simulink model "practia1"  (R2024b)
settings: Solver=VariableStepAuto  StartTime=0.0  StopTime=20  MaxStep=0.01  RelTol=1e-3
InitFcn:
  | ip = 0.0079;
  | Mc = 0.7031;
  | Lp = 0.3302;
  | Mp = 0.23;
  | Fc = 0;
  | Beq = 4.3;
  | g = 9.81;
  | Bp = 0.0024;
settings Model: LastModifiedBy=52332

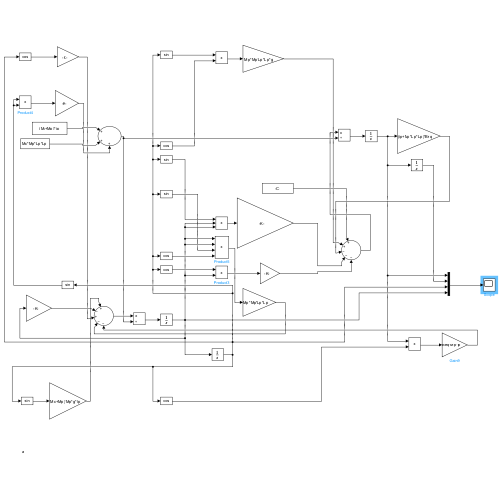
[thumbnail: Simulink's stored preview of the top-level diagram]
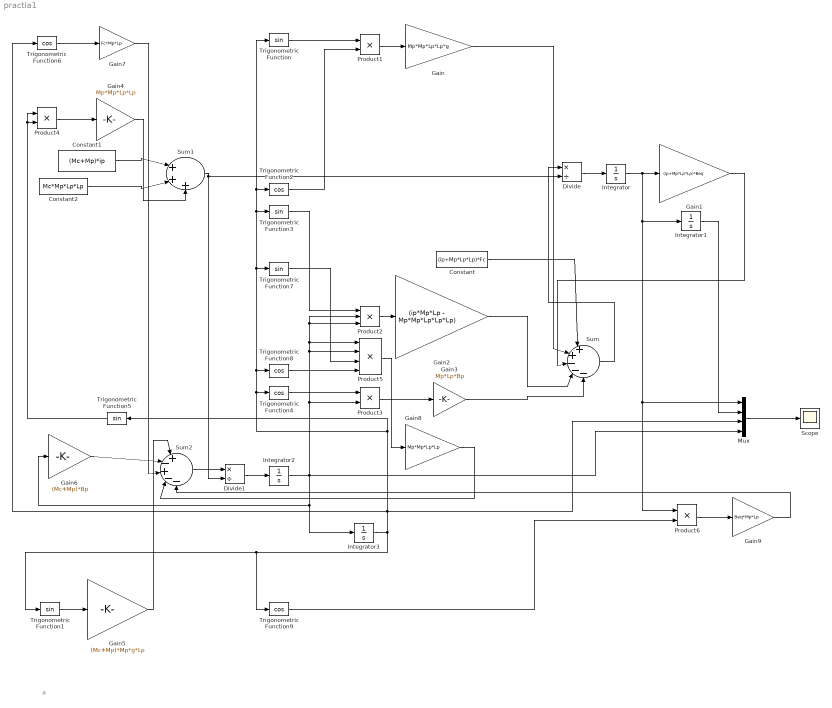
== system practia1 ==
  note: a
  Constant : Constant  Value=(ip+Mp*Lp*Lp)*Fc
  Constant1 : Constant  Value=(Mc+Mp)*ip
  Constant2 : Constant  Value=Mc*Mp*Lp*Lp
  Divide : Product  Inputs=*/
  Divide1 : Product  Inputs=*/
  Gain : Gain  Gain=Mp*Mp*Lp*Lp*g
  Gain1 : Gain  Gain=(ip+Mp*Lp*Lp)*Beq
  Gain2 : Gain  Gain=(ip*Mp*Lp - Mp*Mp*Lp*Lp*Lp)
  Gain3 : Gain  Gain=Mp*Lp*Bp
  Gain4 : Gain  Gain=Mp*Mp*Lp*Lp
  Gain5 : Gain  Gain=(Mc+Mp)*Mp*g*Lp
  Gain6 : Gain  Gain=(Mc+Mp)*Bp
  Gain7 : Gain  Gain=Fc*Mp*Lp
  Gain8 : Gain  Gain=Mp*Mp*Lp*Lp
  Gain9 : Gain  Gain=Beq*Mp*Lp
  Integrator : Integrator
  Integrator1 : Integrator
  Integrator2 : Integrator
  Integrator3 : Integrator  InitialCondition=pi/180
  Mux : Mux
  Product{1,3..4,6} (4 alike) : Product
  Product2 : Product  Inputs=3
  Product5 : Product  Inputs=4
  Scope : Scope
  Sum : Sum  Inputs=|+|+|-|-|-
  Sum1 : Sum  Inputs=|+++
  Sum2 : Sum  Inputs=|+|-|+|-|-
  Trigonometric Function{,1,3,5,7} (5 alike) : Trigonometry
  Trigonometric Function{2,4,6,8..9} (5 alike) : Trigonometry  Operator=cos
  wires:
  Trigonometric Function5/1 -> Product4/1, Product4/2
  Trigonometric Function1/1 -> Gain5/1
  Trigonometric Function6/1 -> Gain7/1
  Sum/1 -> Divide/1
  Product4/1 -> Gain4/1
  Gain4/1 -> Sum1/3
  Divide1/1 -> Integrator2/1
  Gain7/1 -> Sum2/3
  Constant1/1 -> Sum1/1
  Constant2/1 -> Sum1/2
  Gain5/1 -> Sum2/1
  Sum1/1 -> Divide/2, Divide1/2
  Product5/1 -> Gain8/1
  Sum2/1 -> Divide1/1
  Trigonometric Function8/1 -> Product5/4
  Trigonometric Function/1 -> Product1/1
  Trigonometric Function2/1 -> Product1/2
  Trigonometric Function3/1 -> Product2/1
  Trigonometric Function7/1 -> Product5/3
  Trigonometric Function4/1 -> Product3/1
  Integrator2/1 -> Integrator3/1, Gain6/1, Product3/2, Product2/3, Product2/2, Product5/1, Product5/2, Mux/4
  Trigonometric Function9/1 -> Product6/2
  Integrator1/1 -> Mux/2
  Product1/1 -> Gain/1
  Mux/1 -> Scope/1
  Product2/1 -> Gain2/1
  Product3/1 -> Gain3/1
  Integrator3/1 -> Trigonometric Function/1, Trigonometric Function2/1, Trigonometric Function3/1, Trigonometric Function7/1, Trigonometric Function8/1, Trigonometric Function4/1, Trigonometric Function5/1, Trigonometric Function6/1, Mux/3, Trigonometric Function9/1, Trigonometric Function1/1
  Gain6/1 -> Sum2/2
  Gain8/1 -> Sum2/4
  Gain/1 -> Sum/2
  Divide/1 -> Integrator/1
  Constant/1 -> Sum/1
  Gain2/1 -> Sum/4
  Gain3/1 -> Sum/5
  Integrator/1 -> Product6/1, Mux/1, Integrator1/1, Gain1/1
  Gain1/1 -> Sum/3
  Product6/1 -> Gain9/1
  Gain9/1 -> Sum2/5
